simulink model "demo_sys"  (R2023a)
settings: Solver=VariableStepAuto  StartTime=0.0  StopTime=100  RelTol=1e-3
libraries: simulink_extras x1
settings Model: Creator=nikit  LastModifiedBy=nikit

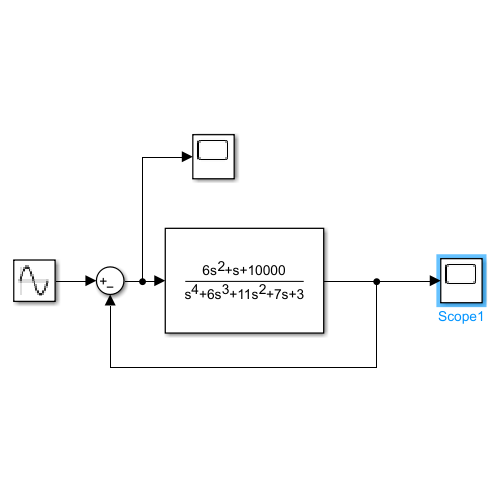
[thumbnail: Simulink's stored preview of the top-level diagram]
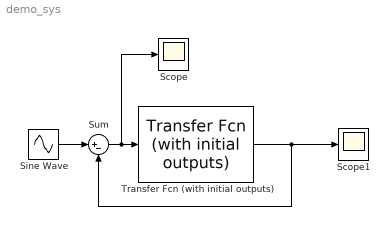
== system demo_sys ==
  Scope : Scope
  Scope1 : Scope
  Sine Wave : Sin  SampleTime=0
  Sum : Sum  Inputs=|+-
  Transfer Fcn (with initial outputs) : simulink_extras/Additional Linear/Transfer Fcn (with initial outputs)  N=[6 1 10000]  D="[1  6 11 7 3]"  Y0=0  U0=0
  wires:
  Sine Wave/1 -> Sum/1
  Sum/1 -> Scope/1, Transfer Fcn (with initial outputs)/1
  Transfer Fcn (with initial outputs)/1 -> Scope1/1, Sum/2
